simulink model "Rocket_Sim_1"  (R2021a)
settings: Solver=VariableStepAuto  StartTime=0.0  StopTime=550  MaxStep=0.001  RelTol=1e-3
values from neighbouring files (symbols this model uses):
  A = (pi*D^2)/4    (= 0.0490873852123)    [init_Rocket_Sim_1.m]    (also in old.m)
  A_drogue = (pi*D_drogue^2)/4    (= 0.125663706144)    [init_Rocket_Sim_1.m]    (also in old.m)
  A_e = pi*(De/2000)^2    (= 0.00196349540849)    [init_Rocket_Sim_1.m]
  A_para = (pi*D_para^2)/4    (= 1.13097335529)    [init_Rocket_Sim_1.m]    (also in old.m)
  Ae = pi*(De/2000)^2    (= 0.00196349540849)    [old.m]
  Cd = 0.5    [init_Rocket_Sim_1.m]    (also in old.m)
  Cd_para = 1.75    [init_Rocket_Sim_1.m]    (also in old.m)
  epsilon = 0.1    [init_Rocket_Sim_1.m]    (also in old.m)
  g = 9.81    [init_Rocket_Sim_1.m]    (also in old.m)
  m_dot = F/V_e    (= 1.78389398573)    [init_Rocket_Sim_1.m]    (also in old.m)
  m_dry = 50    [init_Rocket_Sim_1.m]    (also in old.m)
  m_Propellant = 118    [init_Rocket_Sim_1.m]    (also in old.m)
  p0 = 101325    [init_Rocket_Sim_1.m]    (also in old.m)
  R = 287    [init_Rocket_Sim_1.m]    (also in old.m)
  sigma = 5.6704e-8    (= 5.6704e-08)    [init_Rocket_Sim_1.m]    (also in old.m)
  V_e = g*Isp    (= 1962)    [init_Rocket_Sim_1.m]    (also in suvat_nonsense.m)
  Ve = g*Isp    (= 1962)    [old.m]
undefined symbols (not defined in the file or in its folder): ambient_temp, buck_cout, buck_cout_ESR, Buck_Ilim, buck_ind, buck_ind_ESR, DiscIntNeverNeededParam, Friction, ia, ib, Ion, J, Lithium, Lls, m, m0_fuel, m0_ox, m_f_dot, m_ox_dot, p, Rlim, Rs, supercap_max_voltage, supercap_val, thetam, Ts, Vref, wm
libraries: powerlib x18, electricdrivelib x3, pid_lib x2, powerlib_meascontrol x2, rllib x1
settings Model: SimulationMode=rapid-accelerator  Creator=marti  LastModifiedBy=Raihaan
settings SolverCC: MaxConsecutiveMinStep=5  AlgebraicLoopSolver=TrustRegion
settings DebuggingCC: SFMachineParentedDataDiag=warning

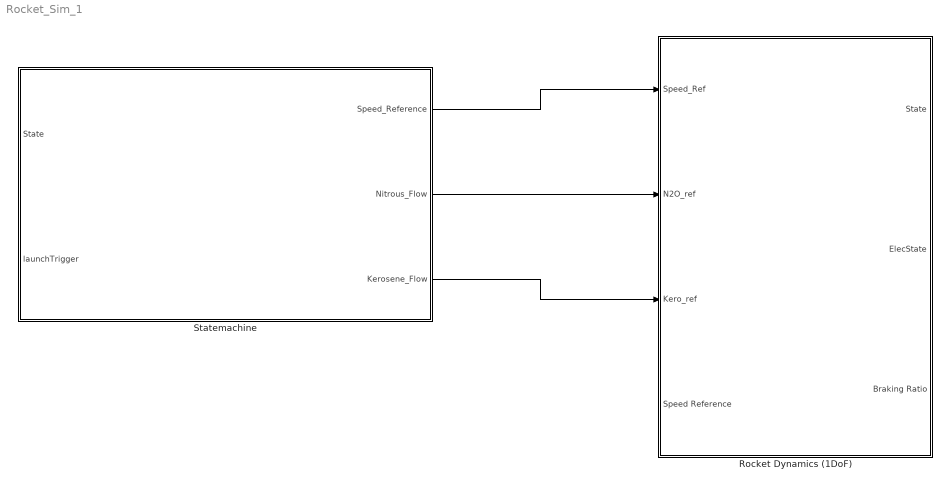
== system Rocket_Sim_1 ==
  Rocket Dynamics (1DoF) : Subsystem
      mask Display: image('$imagefile'); % Use "Edit Image" on toolstrip to change.
  Statemachine : Stateflow chart  TreatAsAtomicUnit=on
  wires:
  Statemachine/1(Speed_Reference) -> Rocket Dynamics (1DoF)/1(Speed_Ref)
  Statemachine/2(Nitrous_Flow) -> Rocket Dynamics (1DoF)/2(N2O_ref)
  Statemachine/3(Kerosene_Flow) -> Rocket Dynamics (1DoF)/3(Kero_ref)

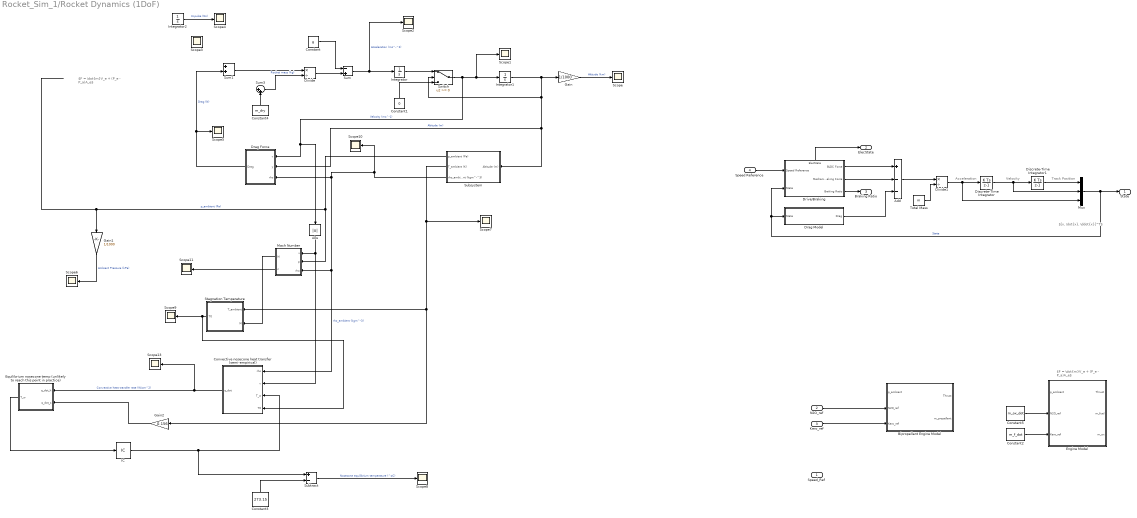
== system Rocket_Sim_1/Rocket Dynamics (1DoF) ==
  note: $F = \dot{m}V_e + (P_e - P_a)A_e$
  note: $[x, \dot{x}, \ddot{x}]^T$
  note: Acceleration
  note: Track Position
  note: Velocity
  note: $F = \dot{m}V_e + (P_e - P_a)A_e$
  Speed_Ref : Inport
  N2O_ref : Inport  Port=2
  Kero_ref : Inport  Port=3
  Speed Reference : Inport  Port=4
  Abs : Abs
  Add : Sum  Inputs=+--
  Bipropellant Engine Model : Subsystem
  Constant : Constant  Value=g
  Constant1 : Constant  Value=0
  Constant2 : Constant  Value=m_f_dot
  Constant3 : Constant  Value=273.15
  Constant4 : Constant  Value=m_dry
  Constant5 : Constant  Value=m_ox_dot
  Convective nosecone heat transfer (semi-empirical) : MATLAB Function  TreatAsAtomicUnit=on
  Discrete-Time Integrator : DiscreteIntegrator  SampleTime=-1  ICPrevOutput=DiscIntNeverNeededParam  ICPrevScaledInput=DiscIntNeverNeededParam
  Discrete-Time Integrator1 : DiscreteIntegrator  SampleTime=-1  LimitOutput=on  UpperSaturationLimit=500  LowerSaturationLimit=0  ICPrevOutput=DiscIntNeverNeededParam  ICPrevScaledInput=DiscIntNeverNeededParam
  Divide : Product  Inputs=*/
  Divide1 : Product  Inputs=*/
  Drag Force : Subsystem
  Drag Model : Subsystem
  Drive/Braking : Subsystem
      settings: PortSchema="{\"entries\":[{\"content\":{\"sides\":[{\"content\":{\"connectorIds\":[\"In1\",\"In2\"]},\"type\":\"ConnectorPlacement.EquallySpacedRectSide\",\"uuid\":\"aa5e316a-c8d3-4f13-ba46-5c76cbb2586c\"},{\"content\":{\"connectorIds\":[\"Out1\",\"Out2\",\"Out3\"],\"side\":\"RIGHT\"},\"type\":\"ConnectorPlacement.EquallySpacedRectSide\",\"uuid\":\"e4d6c32a-fd39-4302-8ddf-f7a48563407f\"},{\"content\":{\"connectorIds\":[\"Out4\"],\"side\":\"TOP\"},\"type\":\"ConnectorPlacement.EquallySpacedRectSide\",\"uuid\":\"af8256cd-30c6-4d91-a38a-bb87ecde33bd\"}]},\"type\":\"ConnectorPlacement.EquallySpacedConnector\",\"uuid\":\"2dd03fee-d1e4-4173-9dcd-593c38e6bfdd\"}],\"packageUris\":[\"http://schema.mathworks.com/mf0/Connector/R2020b\"],\"version\":\"1.0\"}"
  Engine Model : Subsystem
  Equilibrium nosecone temp (unlikely to reach this point in practice) : MATLAB Function  TreatAsAtomicUnit=on
  Gain : Gain  Gain=1/1000
  Gain1 : Gain  Gain=1/1000
  Gain2 : Gain  Gain=0.156
  IC : InitialCondition  Value=300
  Integrator : Integrator
  Integrator1 : Integrator
  Integrator2 : Integrator
  Mach Number : MATLAB Function  TreatAsAtomicUnit=on
  Mux : Mux  Inputs=3
  Scope{,1..11,13} (13 alike) : Scope
  Stagnation Temperature : MATLAB Function  TreatAsAtomicUnit=on
  Subsystem : Subsystem
  Subtract : Sum  Inputs=+-
  Sum : Sum  Inputs=-+
  Sum1 : Sum
  Sum3 : Sum  Inputs=|++
  Switch : Switch
  Total Mass : Constant  Value=m
  State : Outport
  ElecState : Outport  Port=2
  Braking Ratio : Outport  Port=3
  wires:
  Sum/1 -> Scope2/1, Integrator/1  "Acceleration (ms^-^2)"
  Subtract/1 -> Scope8/1  "Nosecone equilibrium temperature (^oC)"
  Constant4/1 -> Sum3/2
  Constant3/1 -> Subtract/2
  Integrator2/1 -> Scope4/1  "Impulse (Ns)"
  Gain1/1 -> Scope6/1  "Ambient Pressure (kPa)"
  Equilibrium nosecone temp (unlikely to reach this point in practice)/1(T_w) -> IC/1
  Integrator/1 -> Switch/1
  Gain2/1 -> Equilibrium nosecone temp (unlikely to reach this point in practice)/2(q_dot_s)
  Constant1/1 -> Switch/3
  Divide/1 -> Sum/2
  IC/1 -> Subtract/1, Convective nosecone heat transfer (semi-empirical)/3(T_w)
  ? -> Sum3/1  "Propellant mass (kg)"
  Abs/1 -> Convective nosecone heat transfer (semi-empirical)/2(v), Mach Number/1(v)
  Subsystem/1(p_ambient (Pa)) -> Mach Number/2(p), Gain1/1  "p_ambient (Pa)"
  Mach Number/1(M) -> Stagnation Temperature/2(M)
  Drag Force/1(Drag) -> Scope5/1, Sum1/2  "Drag (N)"
  Subsystem/3(rho_ambient (kgm^-^3)) -> Scope10/1, Convective nosecone heat transfer (semi-empirical)/1(rho), Mach Number/3(rho), Drag Force/3(rho)  "rho_ambient (kgm^-3)"
  Convective nosecone heat transfer (semi-empirical)/1(q_dot) -> Scope13/1, Equilibrium nosecone temp (unlikely to reach this point in practice)/1(q_dot_h)  "Convective heat transfer rate (W/cm^2)"
  ? -> Integrator2/1, Scope3/1, Sum1/1  "Thrust (N)"
  Switch/1 -> Drag Force/1(v), Abs/1, Scope1/1, Integrator1/1  "Velocity (ms^-1)"
  Sum1/1 -> Divide/1
  Integrator1/1 -> Switch/2, Drag Force/2(y), Subsystem/1(Altitude (m)), Gain/1  "Altitude (m)"
  Sum3/1 -> Divide/2  "Rocket mass (kg)"
  Mach Number/2(c) -> Scope11/1
  Subsystem/2(T_ambient (K)) -> Gain2/1, Stagnation Temperature/1(T_ambient), Scope7/1
  Gain/1 -> Scope/1  "Altitude (km)"
  Constant/1 -> Sum/1
  Stagnation Temperature/1(T0) -> Convective nosecone heat transfer (semi-empirical)/4(T0), Scope9/1
  Discrete-Time Integrator/1 -> Discrete-Time Integrator1/1, Mux/2
  Drag Model/1(Drag) -> Add/3
  Total Mass/1 -> Divide1/2
  Discrete-Time Integrator1/1 -> Mux/1
  Speed Reference/1 -> Drive/Braking/1(Speed Reference)
  Drive/Braking/4(ElecState) -> ElecState/1
  Drive/Braking/1(BLDC Force) -> Add/1
  Drive/Braking/3(Braking Ratio) -> Braking Ratio/1
  Mux/1 -> State/1, Drive/Braking/2(State), Drag Model/1(State)  "State"
  Drive/Braking/2(Mechanical Braking Force) -> Add/2
  Divide1/1 -> Discrete-Time Integrator/1, Mux/3
  Add/1 -> Divide1/1
  Kero_ref/1 -> Bipropellant Engine Model/3(Kero_ref)
  N2O_ref/1 -> Bipropellant Engine Model/2(N2O_ref)
  Constant5/1 -> Engine Model/2(N2O_ref)
  Constant2/1 -> Engine Model/3(Kero_ref)

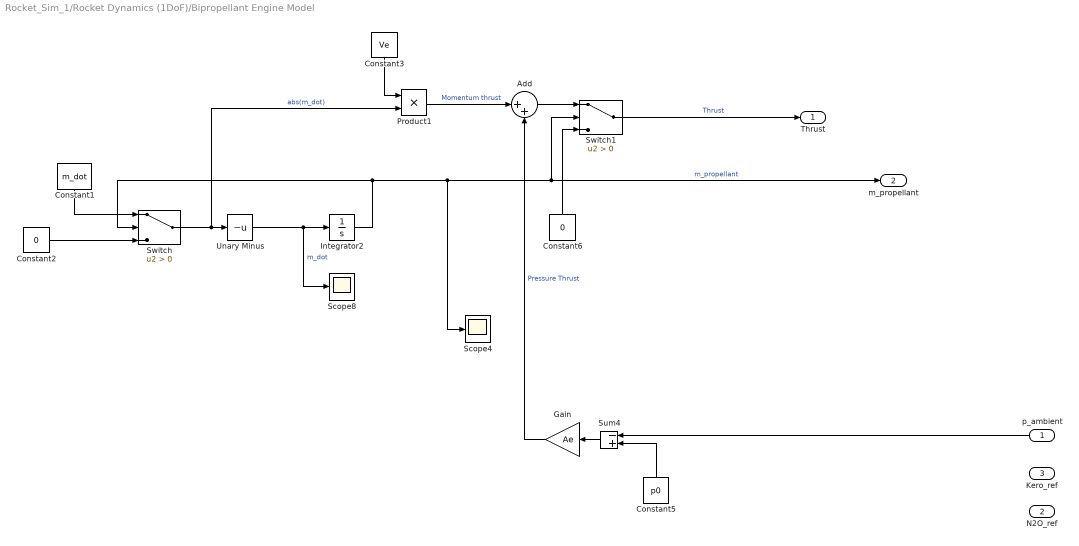
== system Rocket_Sim_1/Rocket Dynamics (1DoF)/Bipropellant Engine Model ==
  p_ambient : Inport
  N2O_ref : Inport  Port=2
  Kero_ref : Inport  Port=3
  Add : Sum  Inputs=|++
  Constant1 : Constant  Value=m_dot
  Constant2 : Constant  Value=0
  Constant3 : Constant  Value=Ve
  Constant5 : Constant  Value=p0
  Constant6 : Constant  Value=0
  Gain : Gain  Gain=Ae
  Integrator2 : Integrator  InitialCondition=m_Propellant
  Product1 : Product
  Scope4 : Scope
  Scope8 : Scope
  Sum4 : Sum  Inputs=-+
  Switch : Switch  Criteria=u2 > Threshold
  Switch1 : Switch  Criteria=u2 > Threshold
  Unary Minus : UnaryMinus
  Thrust : Outport
  m_propellant : Outport  Port=2
  wires:
  Unary Minus/1 -> Integrator2/1, Scope8/1  "m_dot"
  Constant6/1 -> Switch1/3
  Constant2/1 -> Switch/3
  Constant5/1 -> Sum4/2
  Add/1 -> Switch1/1
  Constant3/1 -> Product1/1
  Integrator2/1 -> m_propellant/1, Switch1/2, Scope4/1, Switch/2  "m_propellant"
  Switch/1 -> Product1/2, Unary Minus/1  "abs(m_dot)"
  Sum4/1 -> Gain/1
  Constant1/1 -> Switch/1
  Gain/1 -> Add/2  "Pressure Thrust"
  Switch1/1 -> Thrust/1  "Thrust"
  Product1/1 -> Add/1  "Momentum thrust"
  p_ambient/1 -> Sum4/1

== system Rocket_Sim_1/Rocket Dynamics (1DoF)/Drag Force ==
  v : Inport
  y : Inport  Port=2
  rho : Inport  Port=3
  Drag Force : MATLAB Function  TreatAsAtomicUnit=on
  Switch : Switch
  Unary Minus : UnaryMinus
  Drag : Outport
  wires:
  Drag Force/1(F_d) -> Switch/3, Unary Minus/1  "abs(F_d)"
  Switch/1 -> Drag/1  "F_d"
  v/1 -> Drag Force/1(v), Switch/2
  rho/1 -> Drag Force/3(rho)
  Unary Minus/1 -> Switch/1
  y/1 -> Drag Force/2(y)

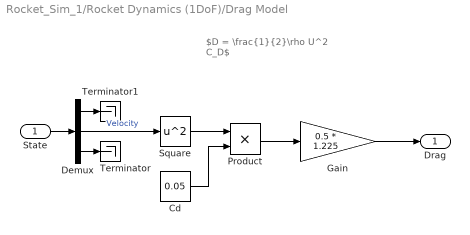
== system Rocket_Sim_1/Rocket Dynamics (1DoF)/Drag Model ==
  note: $D = \frac{1}{2}\rho U^2 C_D$
  State : Inport
  Cd : Constant  Value=0.05
  Demux : Demux  Outputs=3
  Gain : Gain  Gain=0.5 * 1.225
  Product : Product
  Square : Math  Operator=square  SaturateOnIntegerOverflow=on
  Terminator : Terminator
  Terminator1 : Terminator
  Drag : Outport
  wires:
  State/1 -> Demux/1
  Demux/3 -> Terminator/1
  Demux/1 -> Terminator1/1
  Demux/2 -> Square/1  "Velocity"
  Square/1 -> Product/1
  Cd/1 -> Product/2
  Product/1 -> Gain/1
  Gain/1 -> Drag/1

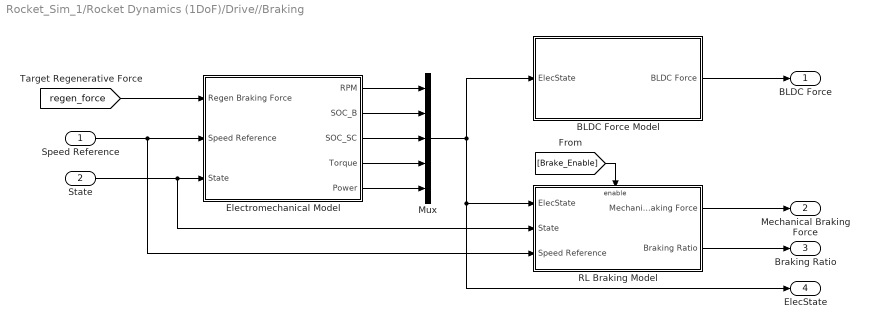
== system Rocket_Sim_1/Rocket Dynamics (1DoF)/Drive//Braking ==
  Speed Reference : Inport
  State : Inport  Port=2
  BLDC Force Model : Subsystem
  Electromechanical Model : Subsystem
  Mux : Mux  Inputs=5
  RL Braking Model : Subsystem
  BLDC Force : Outport
  Mechanical Braking Force : Outport  Port=2
  Braking Ratio : Outport  Port=3
  ElecState : Outport  Port=4
  wires:
  BLDC Force Model/1(BLDC Force) -> BLDC Force/1
  Speed Reference/1 -> Electromechanical Model/2(Speed Reference), RL Braking Model/3(Speed Reference)
  State/1 -> Electromechanical Model/3(State), RL Braking Model/2(State)
  [Brake_Enable] -> RL Braking Model/Enable
  RL Braking Model/2(Braking Ratio) -> Braking Ratio/1
  Electromechanical Model/1(RPM) -> Mux/1
  Electromechanical Model/2(SOC_B) -> Mux/2
  Electromechanical Model/3(SOC_SC) -> Mux/3
  Electromechanical Model/4(Torque) -> Mux/4
  Mux/1 -> ElecState/1, RL Braking Model/1(ElecState), BLDC Force Model/1(ElecState)
  [regen_force] -> Electromechanical Model/1(Regen Braking Force)
  RL Braking Model/1(Mechanical Braking Force) -> Mechanical Braking Force/1
  Electromechanical Model/5(Power) -> Mux/5

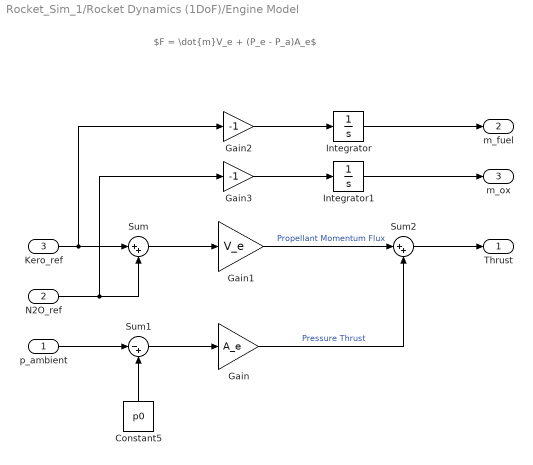
== system Rocket_Sim_1/Rocket Dynamics (1DoF)/Engine Model ==
  note: $F = \dot{m}V_e + (P_e - P_a)A_e$
  p_ambient : Inport
  N2O_ref : Inport  Port=2
  Kero_ref : Inport  Port=3
  Constant5 : Constant  Value=p0
  Gain : Gain  Gain=A_e
  Gain1 : Gain  Gain=V_e
  Gain2 : Gain  Gain=-1
  Gain3 : Gain  Gain=-1
  Integrator : Integrator  InitialCondition=m0_fuel
  Integrator1 : Integrator  InitialCondition=m0_ox
  Sum : Sum  Inputs=|++
  Sum1 : Sum  Inputs=|-+
  Sum2 : Sum  Inputs=|++
  Thrust : Outport
  m_fuel : Outport  Port=2
  m_ox : Outport  Port=3
  wires:
  Kero_ref/1 -> Gain2/1, Sum/1
  N2O_ref/1 -> Sum/2, Gain3/1
  Sum1/1 -> Gain/1
  Sum/1 -> Gain1/1
  Constant5/1 -> Sum1/2
  p_ambient/1 -> Sum1/1
  Gain1/1 -> Sum2/1  "Propellant Momentum Flux"
  Gain/1 -> Sum2/2  "Pressure Thrust"
  Sum2/1 -> Thrust/1
  Integrator/1 -> m_fuel/1
  Gain2/1 -> Integrator/1
  Integrator1/1 -> m_ox/1
  Gain3/1 -> Integrator1/1

== system Rocket_Sim_1/Rocket Dynamics (1DoF)/Subsystem ==
  Altitude (m) : Inport
  Earth Atmosphere Model : MATLAB Function  TreatAsAtomicUnit=on
  p_ambient (Pa) : Outport
  T_ambient (K) : Outport  Port=2
  rho_ambient (kgm^-^3) : Outport  Port=3
  wires:
  Earth Atmosphere Model/1(T) -> T_ambient (K)/1  "T_ambient (K)"
  Altitude (m)/1 -> Earth Atmosphere Model/1(y)
  Earth Atmosphere Model/2(p) -> p_ambient (Pa)/1
  Earth Atmosphere Model/3(rho) -> rho_ambient (kgm^-^3)/1

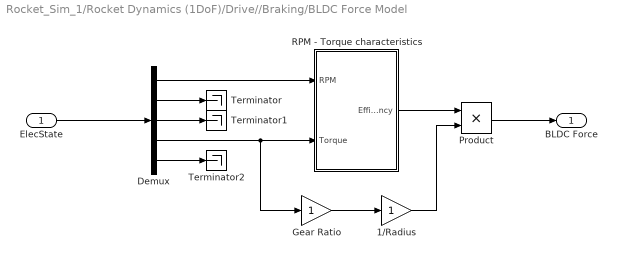
== system Rocket_Sim_1/Rocket Dynamics (1DoF)/Drive//Braking/BLDC Force Model ==
  ElecState : Inport
  1/Radius : Gain
  Demux : Demux  Outputs=5
  Gear Ratio : Gain
  Product : Product
  RPM - Torque characteristics : Subsystem
  Terminator : Terminator
  Terminator1 : Terminator
  Terminator2 : Terminator
  BLDC Force : Outport
  wires:
  Demux/1 -> RPM - Torque characteristics/1(RPM)
  Demux/3 -> Terminator1/1
  Gear Ratio/1 -> 1/Radius/1
  Demux/4 -> RPM - Torque characteristics/2(Torque), Gear Ratio/1
  Product/1 -> BLDC Force/1
  1/Radius/1 -> Product/2
  Demux/2 -> Terminator/1
  ElecState/1 -> Demux/1
  RPM - Torque characteristics/1(Efficiency) -> Product/1
  Demux/5 -> Terminator2/1

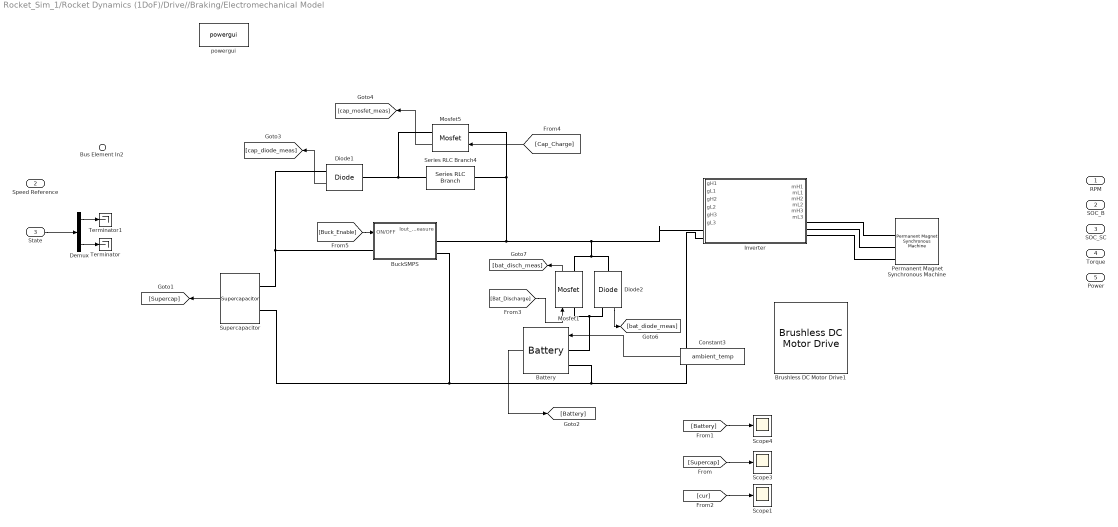
== system Rocket_Sim_1/Rocket Dynamics (1DoF)/Drive//Braking/Electromechanical Model ==
  Bus Element In2 : Inport  PortName=Regen Braking Force  Element=signal1
  Speed Reference : Inport  Port=2
  State : Inport  Port=3
  Battery : electricdrivelib/Extra Sources/Battery  BatType=Lithium-Ion  ShowTempParam=on  ThermalPreset="3.3V  2.3Ah  (LiFePO4)"  ShowAgeParam=off  NomV=3.3  NomQ=2.3  SOC=bat_initial_soc  Batt_Tr=30  PresetModel=off  MaxQ=2.3  MinV=2.475  FullV=3.748  Dis_rate=2.3  R=0.014  Normal_OP=2.25  expZone="[3.4788       0.113]"  current=[6.5 13 32.5]  Units=Time  Tci=20  NomT=25  T2=0  MaxQ2=2.208  FullV2=3.45  Normal_OP2=2.85  expZone2="[3.22       0.015]"  Rca=0.6  ti=1000  Dp=0  Neq0=0  Tsim=1e6  Ta1=25  Qeol=5.4*0.9  Reol=0.013333*1.2  Char_age=[2.3478, 3]  Dis_age=[2.3478, 10]  N1=1500  N2=10500  N3=1000  N4=1400  Ta2=45  N5=950
  Brushless DC Motor Drive1 : electricdrivelib/AC drives/Brushless DC Motor Drive  Rs=0.2  Lls=8.5e-3  Flat=120  MachineConstant=Flux linkage established by magnets (V.s)  FluxCst=0.175  VoltageCst=146.6077  TorqueCst=1.4  ia=0  ib=0  J=0.089  Friction=0.005  p=4  wm=0  thetam=0  Rsnb_rec=10e3  Csnb_rec=20e-9  Ron_rec=1e-3  Vf_rec=1.3  cap_bus=2000e-6  Rbrake=8  fbrake=4000  activationVoltage=320  shutdownVoltage=310  deviceType=IGBT / Diodes  Ron_inv=1e-3  Vf_inv=0.8  Vfd_inv=0.8  Tf=1e-6  Tt=2e-6  Tf_GTO=10e-6  Tt_GTO=20e-6  Rsnb_inv=5000  Csnb_inv=inf  regulationType=Speed regulation  Acc=1000  Dec=-1000  kp_sc=3.3  ki_sc=300  fc_sc=285  Tsc=140e-6  Tmin=-17.8  Tmax=17.8  h=0.01  freq_max=20e3  Tvect=20e-6  zeta=0.99  Trd=0.13/5  K1=3000  K2=-49500  baseSampleTime=2e-06  outputBusMode=Multiple output buses  busLabels=off  sensorless=off  MechanicalLoad=Torque Tm  modelDetailLevel=Detailed  driveType=AC7  AverageValue=off
      settings: SourceProductBaseCode=PS
  BuckSMPS : Subsystem
  Constant3 : Constant  Value=ambient_temp
  Demux : Demux  Outputs=3
  Diode1 : powerlib/Power Electronics/Diode  Ron=0.001  Lon=0  Vf=Vf_Diode  IC=0  UseSnubber=0  Rs=500  Cs=250e-9  Measurements=on
  Diode2 : powerlib/Power Electronics/Diode  Ron=0.001  Lon=0  Vf=Vf_Diode  IC=0  UseSnubber=0  Rs=500  Cs=250e-9  Measurements=on
  Inverter : Subsystem
  Mosfet1 : powerlib/Power Electronics/Mosfet  Ron=Pch_Ron  Lon=0  Rd=0.01  Vfd=Pch_Vd  IC=0  Rs=1e9  Cs=inf  Measurements=on
  Mosfet5 : powerlib/Power Electronics/Mosfet  Ron=Pch_Ron  Lon=0  Rd=0.01  Vfd=Pch_Vd  IC=0  Rs=1e9  Cs=inf  Measurements=on
  Permanent Magnet Synchronous Machine : powerlib/Machines/Permanent Magnet Synchronous Machine  NbPhases=3  FluxDistribution=Trapezoidal  RotorType=Round  MechanicalLoad=Torque Tm  PresetModel=No  ShowDetailedParameters=on  MeasurementBus=off  Resistance=Rs  Inductance=Lls  dqInductances=[8.5e-3,8.5e-3]  La=0.000835  MachineConstant=Flux linkage established by magnets (V.s)  Flux=0.175  VoltageCst=146.6077  TorqueCst=1.4  Flat=Flat  Mechanical=[J,Friction,p]  PolePairs=4  InitialConditions=[wm,thetam,ia,ib]  InitialConditions5ph=[0 0 0 0 0 0]  RefAngle=90 degrees behind phase A axis (modified Park)  IterativeDiscreteModel=Trapezoidal non iterative  TsBlock=-1  TsPowergui=0
  Scope1 : Scope
  Scope3 : Scope
  Scope4 : Scope
  Series RLC Branch4 : powerlib/Elements/Series RLC Branch  LConnTagsString=__new0  RConnTagsString=__new0  BranchType=R  Resistance=Rlim  Inductance=1e-3  SetiL0=off  InitialCurrent=0  Capacitance=1e-6  Setx0=off  InitialVoltage=0  Measurements=Branch voltage and current
  Supercapacitor : electricdrivelib/Extra Sources/Supercapacitor  C=supercap_val  Rdc=supercap_ESR  Voltage=supercap_max_voltage  Ns=18  Np=1  Vinit=supercap_initial_voltage  Temp=ambient_temp  PresetModel=off  EstParam=off  Nc=1  r=1e-9  epsilon=6.0208e-10  Ich=10  Vstern="[0.161  2.7  7.8]"  Self_dis=on  Ioc=10  Vself="[48  47.8  47.06  44.65]"  demandeplot=off  I="[10  20 100  500]"  Units=sec  Vmax=0  If=0  deltaV=0  alpha=0  sec=0
      settings: SourceProductBaseCode=PS
  Terminator : Terminator
  Terminator1 : Terminator
  powergui : powerlib/powergui  Priority=1  SimulationMode=Discrete  SampleTime=Ts  frequency=60  Iterations=50  frequencyindice=0  Pbase=100e6  ErrMax=1e-4  UnitsV=kV  UnitsW=MW  buscounter=0  FunctionMessages=off  echomessages=off  EnableUseOfTLC=off  CurrentSourceSwitches=off  DisableSnubberDevices=off  DisableRonSwitches=off  DisableVfSwitches=off  DisplayEquations=off  AutomaticDiscreteSolvers=off  SolverType=Tustin/Backward Euler (TBE)  Interpol=off  ExternalGateDelay=off  methode=off  Ts=100  x0status=blocks  SPID=on  SwTol=0  HookPort=off  NonlinearTolerance=1e-4  nMaxIteration=100  ContinueOnMaxIteration=off  RestoreLinks=warning  ResistiveCurrentMeasurement=off  Frange=[0:2:500]  Ylog=off  Xlog=on  ShowGrid=off  save=off  variable=ZData  structure=0  ZoomFFT=off  StartTime=0.0  cycles=1  DisplayStyle=1  fundamental=60  FreqAxis=off  MaxFrequency=1000  frequencyindicesteady=1  RmsSteady=1  display=off
  RPM : Outport
  SOC_B : Outport  Port=2
  SOC_SC : Outport  Port=3
  Torque : Outport  Port=4
  Power : Outport  Port=5
  wires:
  [Battery] -> Scope4/1
  [cur] -> Scope1/1
  Diode2/1 -> [bat_diode_meas]
  [Cap_Charge] -> Mosfet5/1
  Mosfet5/1 -> [cap_mosfet_meas]
  Mosfet1/1 -> [bat_disch_meas]
  Battery/1 -> [Battery]
  Diode1/1 -> [cap_diode_meas]
  Constant3/1 -> Battery/1
  Supercapacitor/1 -> [Supercap]
  [Supercap] -> Scope3/1
  Demux/1 -> Terminator1/1
  Demux/3 -> Terminator/1
  State/1 -> Demux/1
  [Bat_Discharge] -> Mosfet1/1
  [Buck_Enable] -> BuckSMPS/1(ON/OFF)
  connections:
  Series RLC Branch4/LConn1 -- Mosfet1/RConn1 -- Diode2/LConn1 -- Inverter/LConn1 -- BuckSMPS/RConn1 -- Mosfet5/LConn1
  Diode1/RConn1 -- BuckSMPS/LConn1 -- Supercapacitor/LConn1
  Inverter/LConn2 -- BuckSMPS/RConn2 -- Supercapacitor/LConn2 -- Battery/LConn2
  Mosfet1/LConn1 -- Diode2/RConn1 -- Battery/LConn1
  Diode1/LConn1 -- Series RLC Branch4/RConn1 -- Mosfet5/RConn1
  Inverter/RConn3 -- Permanent Magnet Synchronous Machine/LConn3
  Permanent Magnet Synchronous Machine/LConn1 -- Inverter/RConn1
  Inverter/RConn2 -- Permanent Magnet Synchronous Machine/LConn2

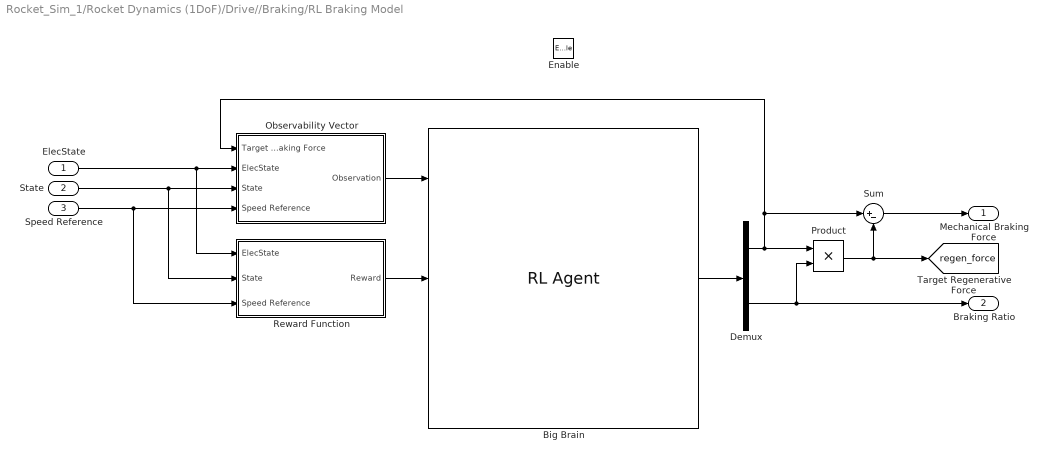
== system Rocket_Sim_1/Rocket Dynamics (1DoF)/Drive//Braking/RL Braking Model ==
  ElecState : Inport
  State : Inport  Port=2
  Speed Reference : Inport  Port=3
  Enable : EnablePort
  Big Brain : rllib/RL Agent  Agent=agentObj  ExternalActionAsInput=off  ProvideCumRwd=off  TreatAsDirectFeedthrough=on  mask(RL Agent){}
      mask Display: image('$imagefile'); % Use "Edit Image" on toolstrip to change.
  Demux : Demux  Outputs=2
  Observability Vector : Subsystem
      mask Display: image('$imagefile'); % Use "Edit Image" on toolstrip to change.
  Product : Product
  Reward Function : Subsystem
      mask Display: image('$imagefile'); % Use "Edit Image" on toolstrip to change.
  Sum : Sum  Inputs=|+-
  Mechanical Braking Force : Outport
  Braking Ratio : Outport  Port=2
  tag scope: regen_force=global
  wires:
  State/1 -> Reward Function/2(State), Observability Vector/3(State)
  Reward Function/1(Reward) -> Big Brain/2
  Observability Vector/1(Observation) -> Big Brain/1
  ElecState/1 -> Reward Function/1(ElecState), Observability Vector/2(ElecState)
  Product/1 -> Sum/2, [regen_force]
  Big Brain/1 -> Demux/1
  Demux/1 -> Product/1, Observability Vector/1(Target Braking Force), Sum/1
  Demux/2 -> Product/2, Braking Ratio/1
  Speed Reference/1 -> Reward Function/3("Speed Reference "), Observability Vector/4(Speed Reference)
  Sum/1 -> Mechanical Braking Force/1

== system Rocket_Sim_1/Rocket Dynamics (1DoF)/Drive//Braking/BLDC Force Model/RPM - Torque characteristics ==
  RPM : Inport
  Torque : Inport  Port=2
  Gain : Gain
  Efficiency : Outport
  wires:
  RPM/1 -> Gain/1
  Gain/1 -> Efficiency/1

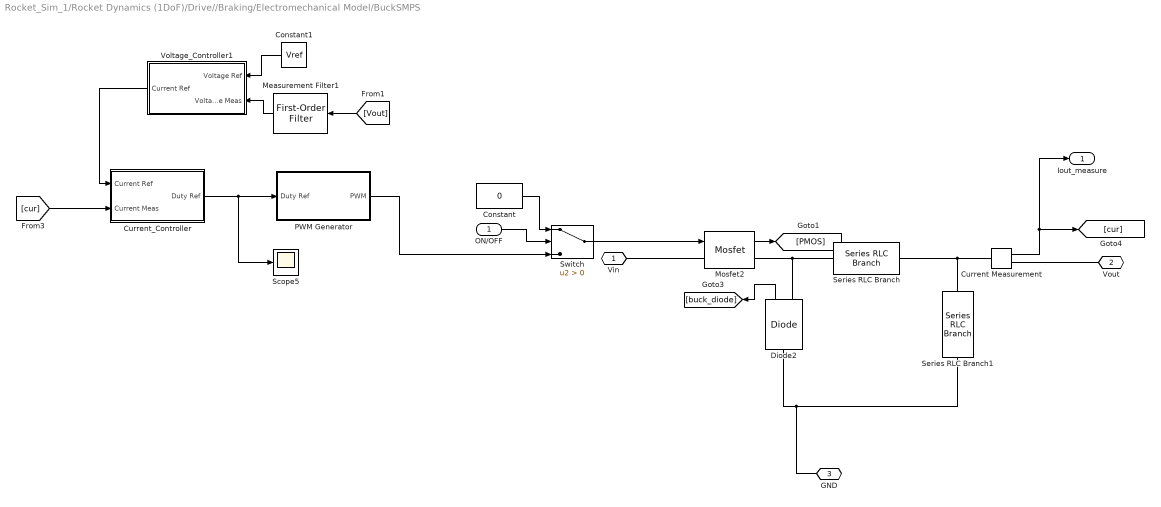
== system Rocket_Sim_1/Rocket Dynamics (1DoF)/Drive//Braking/Electromechanical Model/BuckSMPS ==
  ON/OFF : Inport
  Constant : Constant  Value=0
  Constant1 : Constant  Value=Vref
  Current Measurement : powerlib/Measurements/Current Measurement  PhasorSimulation=off  OutputType=Complex  PSBequivalent=0
  Current_Controller : Subsystem
  Diode2 : powerlib/Power Electronics/Diode  Ron=0.001  Lon=0  Vf=Vf_Diode  IC=0  UseSnubber=0  Rs=500  Cs=250e-9  Measurements=on
  Measurement Filter1 : powerlib_meascontrol/Filters/First-Order Filter  FilterType=Lowpass  Tc=10000*2.2e-9  Ts=0  Initialize=on  Vac_Init=[0, 0, 0]  Vdc_Init=0  PlotResponse=off  FreqRange="[0,  100e3,  100]"
  Mosfet2 : powerlib/Power Electronics/Mosfet  Ron=Pch_Ron  Lon=0  Rd=0.01  Vfd=Pch_Vd  IC=0  Rs=1e9  Cs=inf  Measurements=on
  PWM Generator : Subsystem
  Scope5 : Scope
  Series RLC Branch : powerlib/Elements/Series RLC Branch  LConnTagsString=__new0  RConnTagsString=__new0  BranchType=RL  Resistance=buck_ind_ESR  Inductance=buck_ind  SetiL0=off  InitialCurrent=0  Capacitance=1e-6  Setx0=off  InitialVoltage=0  Measurements=None
  Series RLC Branch1 : powerlib/Elements/Series RLC Branch  LConnTagsString=__new0  RConnTagsString=__new0  BranchType=RC  Resistance=buck_cout_ESR  Inductance=1e-3  SetiL0=off  InitialCurrent=0  Capacitance=buck_cout  Setx0=off  InitialVoltage=0  Measurements=Branch voltage and current
  Switch : Switch  Criteria=u2 > Threshold
  Voltage_Controller1 : Subsystem
  Vin : PMIOPort  Side=Left
  Vout : PMIOPort  Port=2  Side=Right
  GND : PMIOPort  Port=3  Side=Right
  Iout_measure : Outport
  wires:
  [cur] -> Current_Controller/2(Current Meas)
  PWM Generator/1(PWM) -> Switch/3
  Current Measurement/1 -> Iout_measure/1, [cur]
  Current_Controller/1(Duty Ref) -> Scope5/1, PWM Generator/1(Duty Ref)
  Mosfet2/1 -> [PMOS]
  Diode2/1 -> [buck_diode]
  [Vout] -> Measurement Filter1/1
  Measurement Filter1/1 -> Voltage_Controller1/2(Voltage Meas)
  Constant1/1 -> Voltage_Controller1/1(Voltage Ref)
  Voltage_Controller1/1(Current Ref) -> Current_Controller/1(Current Ref)
  ON/OFF/1 -> Switch/2
  Switch/1 -> Mosfet2/1
  Constant/1 -> Switch/1
  connections:
  Mosfet2/RConn1 -- Diode2/RConn1 -- Series RLC Branch/LConn1
  Series RLC Branch/RConn1 -- Current Measurement/LConn1 -- Series RLC Branch1/LConn1
  Current Measurement/RConn1 -- Vout/RConn1
  Mosfet2/LConn1 -- Vin/RConn1
  Series RLC Branch1/RConn1 -- Diode2/LConn1 -- GND/RConn1

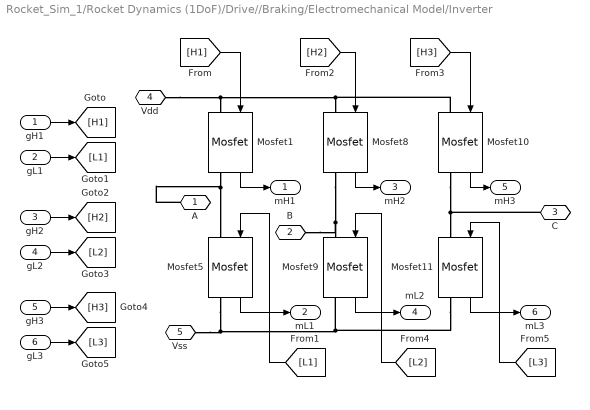
== system Rocket_Sim_1/Rocket Dynamics (1DoF)/Drive//Braking/Electromechanical Model/Inverter ==
  gH1 : Inport
  gL1 : Inport  Port=2
  gH2 : Inport  Port=3
  gL2 : Inport  Port=4
  gH3 : Inport  Port=5
  gL3 : Inport  Port=6
  Mosfet{1,5,8..11} (6 alike) : powerlib/Power Electronics/Mosfet  Ron=0.1  Lon=0  Rd=0.01  Vfd=0  IC=0  Rs=1e5  Cs=inf  Measurements=on
  A : PMIOPort  Side=Right
  B : PMIOPort  Port=2  Side=Right
  C : PMIOPort  Port=3  Side=Right
  Vdd : PMIOPort  Port=4  Side=Left
  Vss : PMIOPort  Port=5  Side=Left
  mH1 : Outport
  mL1 : Outport  Port=2
  mH2 : Outport  Port=3
  mL2 : Outport  Port=4
  mH3 : Outport  Port=5
  mL3 : Outport  Port=6
  wires:
  Mosfet11/1 -> mL3/1
  [L2] -> Mosfet9/1
  Mosfet5/1 -> mL1/1
  [H3] -> Mosfet10/1
  gL2/1 -> [L2]
  [H2] -> Mosfet8/1
  Mosfet9/1 -> mL2/1
  Mosfet10/1 -> mH3/1
  Mosfet1/1 -> mH1/1
  Mosfet8/1 -> mH2/1
  [L1] -> Mosfet5/1
  gL3/1 -> [L3]
  gH3/1 -> [H3]
  gL1/1 -> [L1]
  gH2/1 -> [H2]
  gH1/1 -> [H1]
  [H1] -> Mosfet1/1
  [L3] -> Mosfet11/1
  connections:
  Mosfet5/RConn1 -- Vss/RConn1 -- Mosfet11/RConn1 -- Mosfet9/RConn1
  Vdd/RConn1 -- Mosfet8/LConn1 -- Mosfet10/LConn1 -- Mosfet1/LConn1
  Mosfet1/RConn1 -- Mosfet5/LConn1 -- A/RConn1
  Mosfet10/RConn1 -- Mosfet11/LConn1 -- C/RConn1
  Mosfet8/RConn1 -- B/RConn1 -- Mosfet9/LConn1

== system Rocket_Sim_1/Rocket Dynamics (1DoF)/Drive//Braking/RL Braking Model/Observability Vector ==
  Target Braking Force : Inport
  ElecState : Inport  Port=2
  State : Inport  Port=3
  Speed Reference : Inport  Port=4
  Mux : Mux
  Observation : Outport
  wires:
  Mux/1 -> Observation/1
  Target Braking Force/1 -> Mux/1
  ElecState/1 -> Mux/2
  State/1 -> Mux/3
  Speed Reference/1 -> Mux/4

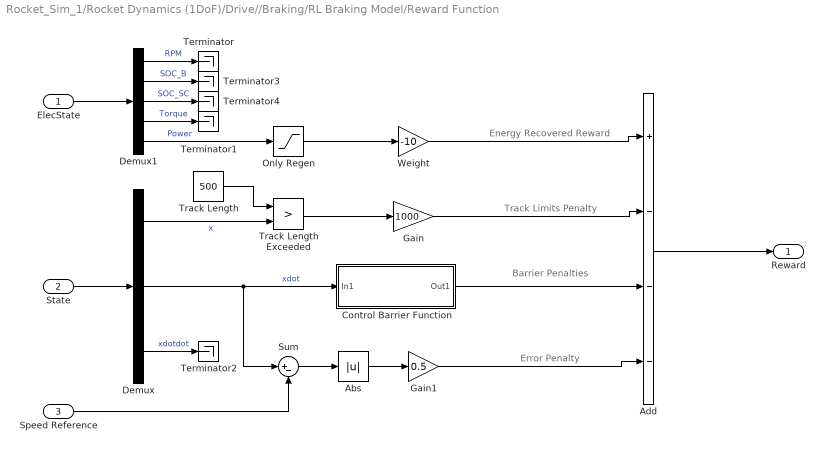
== system Rocket_Sim_1/Rocket Dynamics (1DoF)/Drive//Braking/RL Braking Model/Reward Function ==
  note: Barrier Penalties
  note: Track Limits Penalty
  note: Error Penalty
  note: Energy Recovered Reward
  ElecState : Inport
  State : Inport  Port=2
  "Speed Reference " : Inport  Port=3
  Abs : Abs
  Add : Sum  Inputs=+---
  Control Barrier Function : Subsystem
  Demux : Demux  Outputs=3
  Demux1 : Demux  Outputs=5
  Gain : Gain  Gain=1000
  Gain1 : Gain  Gain=0.5
  Only Regen : Saturate  UpperLimit=0  LowerLimit=-inf
  Sum : Sum  Inputs=|+-
  Terminator{,1..4} (5 alike) : Terminator
  Track Length : Constant  Value=500
  Track Length Exceeded : RelationalOperator  Operator=>  OutDataTypeStr=boolean  RndMeth=Simplest
  Weight : Gain  Gain=-10
  Reward : Outport
  wires:
  Demux1/3 -> Terminator4/1  "SOC_SC"
  Demux/1 -> Track Length Exceeded/2  "x"
  Abs/1 -> Gain1/1
  Sum/1 -> Abs/1
  Track Length Exceeded/1 -> Gain/1
  Gain1/1 -> Add/4
  Gain/1 -> Add/2
  "Speed Reference "/1 -> Sum/2
  Weight/1 -> Add/1
  Track Length/1 -> Track Length Exceeded/1
  Demux/2 -> Sum/1, Control Barrier Function/1(In1)  "xdot"
  Control Barrier Function/1(Out1) -> Add/3
  Only Regen/1 -> Weight/1
  State/1 -> Demux/1
  Demux/3 -> Terminator2/1  "xdotdot"
  Demux1/1 -> Terminator/1  "RPM"
  ElecState/1 -> Demux1/1
  Demux1/4 -> Terminator1/1  "Torque"
  Demux1/5 -> Only Regen/1  "Power"
  Add/1 -> Reward/1
  Demux1/2 -> Terminator3/1  "SOC_B"

== system Rocket_Sim_1/Rocket Dynamics (1DoF)/Drive//Braking/Electromechanical Model/BuckSMPS/Current_Controller ==
  Current Ref : Inport
  Current Meas : Inport  Port=2
  Discrete PID Controller : pid_lib/PID Controller  Controller=PID  Form=Parallel  TimeDomain=Discrete-time  UseExternalTs=off  SampleTime=1/1000  IntegratorMethod=Forward Euler  FilterMethod=Forward Euler  ControllerParametersSource=internal  P=0.02512  I=39.4  D=0  UseFilter=off  N=100  TunerSelectOption=Transfer Function Based (PID Tuner App)  InitialConditionSource=internal  InitialConditionForIntegrator=0  InitialConditionForFilter=0  DifferentiatorICPrevScaledInput=0  ExternalReset=none  TrackingMode=off  Kt=1  LimitOutput=off  SatLimitsSource=internal  UpperSaturationLimit=inf  LowerSaturationLimit=-inf  LinearizeAsGain=off  AntiWindupMode=none  Kb=1  POutMin=[]  POutMax=[]  IOutMin=[]  IOutMax=[]  DOutMin=[]  DOutMax=[]  NOutMin=[]  NOutMax=[]  SumOutMin=[]  SumOutMax=[]  SaturationOutMin=[]  SaturationOutMax=[]  PParamMin=[]  PParamMax=[]  IParamMin=[]  IParamMax=[]  DParamMin=[]  DParamMax=[]  NParamMin=[]  NParamMax=[]  KbParamMin=[]  KbParamMax=[]  KtParamMin=[]  KtParamMax=[]  KbOutMin=[]  KbOutMax=[]  KtOutMin=[]  KtOutMax=[]  IntegratorOutMin=[]  IntegratorOutMax=[]  FilterOutMin=[]  FilterOutMax=[]  SumI1OutMin=[]  SumI1OutMax=[]  SumI2OutMin=[]  SumI2OutMax=[]  SumI3OutMin=[]  SumI3OutMax=[]  SumI4OutMin=[]  SumI4OutMax=[]  SumDOutMin=[]  SumDOutMax=[]  DifferentiatorOutMin=[]  DifferentiatorOutMax=[]  FilterDiffOutCoefMin=[]  FilterDiffOutCoefMax=[]  ReciprocalOutMin=[]  ReciprocalOutMax=[]  SumDenOutMin=[]  SumDenOutMax=[]  SumNumOutMin=[]  SumNumOutMax=[]  DivideOutMin=[]  DivideOutMax=[]  UdiffTsProdOutMin=[]  UdiffTsProdOutMax=[]  NTsProdOutMin=[]  NTsProdOutMax=[]  UintegralTsProdOutMin=[]  UintegralTsProdOutMax=[]  UngainTsProdOutMin=[]  UngainTsProdOutMax=[]  IntegratorContinuousStateAttributes=''  IntegratorStateMustResolveToSignalObject=off  IntegratorRTWStateStorageClass=Auto  FilterContinuousStateAttributes=''  FilterStateMustResolveToSignalObject=off  FilterRTWStateStorageClass=Auto  ParallelPVariant=InternalParameters  IdealPVariant=Disabled  IVariant=InternalParameters  DVariant=InternalParameters  IntegratorVariant=Discrete  SatVariant=Disabled  AWVariant=Passthrough  PCopyVariant=Disabled  TRVariant=Disabled  FdbkBlocksVariant=Forward  IdealPFdbkVariant=Disabled  SatFdbkVariant=Disabled  DerivativeFilterVariant=Differentiator  NVariant=Passthrough  NCopyVariant=Disabled_SignalSpec  FilterICVariant=InternalICsDifferentiator  IntegratorICVariant=InternalICs  ExternalResetVariant=Disabled  TRSumVariant=Passthrough  SumFdbkVariant=Disabled  SumVariant=Sum_PID  TsampFilterVariant=InternalTs  TsampNgainVariant=Passthrough  TsampIntegralVariant=Passthrough  ExternalSaturationOutDataTypeStr=Inherit: Same as second input
  Saturation : Saturate  UpperLimit=0.98  LowerLimit=0.02
  Subtract : Sum  Inputs=+-
  Duty Ref : Outport
  wires:
  Subtract/1 -> Discrete PID Controller/1
  Saturation/1 -> Duty Ref/1
  Current Meas/1 -> Subtract/2
  Discrete PID Controller/1 -> Saturation/1
  Current Ref/1 -> Subtract/1

== system Rocket_Sim_1/Rocket Dynamics (1DoF)/Drive//Braking/Electromechanical Model/BuckSMPS/PWM Generator ==
  note: This is a PWM generator using a sawtooth waveform and comparator.
      |
      | The sawtooth function gives an output +/-1 and we need to be in the range 0-1 and therefore needs offsetting.
  Duty Ref : Inport
  Add : Sum
  Constant : Constant
  Gain : Gain  Gain=0.5
  Relational Operator : RelationalOperator  Operator=>  OutDataTypeStr=boolean  RndMeth=Simplest
  Sawtooth Generator : powerlib_meascontrol/Pulse & Signal Generators/Sawtooth Generator  Freq=62500  Phase=180  Ts=Ts
  PWM : Outport
  wires:
  Duty Ref/1 -> Relational Operator/1
  Relational Operator/1 -> PWM/1
  Constant/1 -> Add/2
  Add/1 -> Gain/1
  Sawtooth Generator/1 -> Add/1
  Gain/1 -> Relational Operator/2

== system Rocket_Sim_1/Rocket Dynamics (1DoF)/Drive//Braking/Electromechanical Model/BuckSMPS/Voltage_Controller1 ==
  Voltage Ref : Inport
  Voltage Meas : Inport  Port=2
  Discrete PID Controller1 : pid_lib/PID Controller  Controller=PID  Form=Parallel  TimeDomain=Discrete-time  UseExternalTs=off  SampleTime=1/1000  IntegratorMethod=Forward Euler  FilterMethod=Forward Euler  ControllerParametersSource=internal  P=0.05024  I=15.78  D=0  UseFilter=off  N=100  TunerSelectOption=Transfer Function Based (PID Tuner App)  InitialConditionSource=internal  InitialConditionForIntegrator=0  InitialConditionForFilter=0  DifferentiatorICPrevScaledInput=0  ExternalReset=none  TrackingMode=off  Kt=1  LimitOutput=off  SatLimitsSource=internal  UpperSaturationLimit=inf  LowerSaturationLimit=-inf  LinearizeAsGain=off  AntiWindupMode=none  Kb=1  POutMin=[]  POutMax=[]  IOutMin=[]  IOutMax=[]  DOutMin=[]  DOutMax=[]  NOutMin=[]  NOutMax=[]  SumOutMin=[]  SumOutMax=[]  SaturationOutMin=[]  SaturationOutMax=[]  PParamMin=[]  PParamMax=[]  IParamMin=[]  IParamMax=[]  DParamMin=[]  DParamMax=[]  NParamMin=[]  NParamMax=[]  KbParamMin=[]  KbParamMax=[]  KtParamMin=[]  KtParamMax=[]  KbOutMin=[]  KbOutMax=[]  KtOutMin=[]  KtOutMax=[]  IntegratorOutMin=[]  IntegratorOutMax=[]  FilterOutMin=[]  FilterOutMax=[]  SumI1OutMin=[]  SumI1OutMax=[]  SumI2OutMin=[]  SumI2OutMax=[]  SumI3OutMin=[]  SumI3OutMax=[]  SumI4OutMin=[]  SumI4OutMax=[]  SumDOutMin=[]  SumDOutMax=[]  DifferentiatorOutMin=[]  DifferentiatorOutMax=[]  FilterDiffOutCoefMin=[]  FilterDiffOutCoefMax=[]  ReciprocalOutMin=[]  ReciprocalOutMax=[]  SumDenOutMin=[]  SumDenOutMax=[]  SumNumOutMin=[]  SumNumOutMax=[]  DivideOutMin=[]  DivideOutMax=[]  UdiffTsProdOutMin=[]  UdiffTsProdOutMax=[]  NTsProdOutMin=[]  NTsProdOutMax=[]  UintegralTsProdOutMin=[]  UintegralTsProdOutMax=[]  UngainTsProdOutMin=[]  UngainTsProdOutMax=[]  IntegratorContinuousStateAttributes=''  IntegratorStateMustResolveToSignalObject=off  IntegratorRTWStateStorageClass=Auto  FilterContinuousStateAttributes=''  FilterStateMustResolveToSignalObject=off  FilterRTWStateStorageClass=Auto  ParallelPVariant=InternalParameters  IdealPVariant=Disabled  IVariant=InternalParameters  DVariant=InternalParameters  IntegratorVariant=Discrete  SatVariant=Disabled  AWVariant=Passthrough  PCopyVariant=Disabled  TRVariant=Disabled  FdbkBlocksVariant=Forward  IdealPFdbkVariant=Disabled  SatFdbkVariant=Disabled  DerivativeFilterVariant=Differentiator  NVariant=Passthrough  NCopyVariant=Disabled_SignalSpec  FilterICVariant=InternalICsDifferentiator  IntegratorICVariant=InternalICs  ExternalResetVariant=Disabled  TRSumVariant=Passthrough  SumFdbkVariant=Disabled  SumVariant=Sum_PID  TsampFilterVariant=InternalTs  TsampNgainVariant=Passthrough  TsampIntegralVariant=Passthrough  ExternalSaturationOutDataTypeStr=Inherit: Same as second input
  Saturation1 : Saturate  UpperLimit=Buck_Ilim  LowerLimit=0
  Subtract1 : Sum  Inputs=+-
  Current Ref : Outport
  wires:
  Saturation1/1 -> Current Ref/1
  Subtract1/1 -> Discrete PID Controller1/1
  Voltage Ref/1 -> Subtract1/1
  Discrete PID Controller1/1 -> Saturation1/1
  Voltage Meas/1 -> Subtract1/2

== system Rocket_Sim_1/Rocket Dynamics (1DoF)/Drive//Braking/RL Braking Model/Reward Function/Control Barrier Function ==
  In1 : Inport
  Out1 : Outport
  wires:
  In1/1 -> Out1/1

== matlab function Rocket_Sim_1/Rocket Dynamics (1DoF)/Drag Force/Drag Force ==
  data: v input; y input; F_d output; rho input; Cd parameter; A parameter; Cd_para parameter; A_para parameter; A_drogue parameter
function F_d = fcn(v, y, rho, Cd, A, Cd_para, A_para, A_drogue)
if v > -20
    F_d = 0.5*A*rho*Cd*v^2; %Calculate drag force for rocket on ascent
else
    if y > 1000
        F_d = 0.5*A*rho*Cd*v^2 + 0.5*A_drogue*rho*Cd_para*v^2; %Calculate drag force for rocket + drogue parachute on descent
    elseif y >800
        F_d = 0.5*A*rho*Cd*v^2 + 0.5*(A_para/2)*rho*Cd_para*v^2; %Calculate drag force for rocket + reefed parachute on descent
    else
        F_d = 0.5*A*rho*Cd*v^2 + 0.5*A_para*rho*Cd_para*v^2; %Calculate drag force for rocket + parachute on descent
    end
end

== matlab function Rocket_Sim_1/Rocket Dynamics (1DoF)/Subsystem/Earth Atmosphere Model ==
  data: y input; T output; p output; rho output; p0 parameter; R parameter; g parameter
function [T, p, rho] = fcn(y, p0, R, g)
%Using NASA atmosphere model for pressure: https://www.grc.nasa.gov/www/k-12/airplane/atmosmet.html
%And "definition of standard temperatures at different altitudes" for temperature: http://www.ambrsoft.com/CalcPhysics/Altitude/altitude.htm

T0 = 288.15; %Temperature at y = 0
L0 = -0.0065; %Rate of change of temperature with height (in K/m)

T1 = 216.65;
p1 = p0*(T1/T0)^(-g/(R*L0));

T2 = T1;
L2 = 0.001;
p2 = p1*exp(g*(11000 - 20000)/(R*T2));

T3 = 228.65;
L3 = 0.0028;
p3 = p2*(T3/T2)^(-g/(R*L2));

T4 = 270.65;
p4 = p3*(T4/T3)^(-g/(R*L3));

T5 = T4;
L5 = -0.0028;
p5 = p4*exp(g*(47000 - 51000)/(R*T4));

T6 = 214.65;
L6 = -0.002;
p6 = p5*(T6/T5)^(-g/(R*L5));

T7 = 186.95;
p7 = p6*(T7/T6)^(-g/(R*L6));

T8 = T7;
L8 = 0.004;
p8 = p7*exp(g*(84852 - 90000)/(R*T7));

%Work out atmospheric temperature in K
if y < 11000 %Troposphere (0 to 1)
    T = T0 + L0*y;
    p = p0*(T/T0)^(-g/(R*L0));
elseif y >= 11000 && y < 20000 %Tropopause (1 to 2)
    T = T1;
    p = p1*exp(g*(11000 - y)/(R*T1));
elseif y >= 20000 && y < 32000 %Lower stratosphere (2 to 3)
    T = T2 + L2*(y - 20000);
    p = p2*(T/T2)^(-g/(R*L2));
elseif y >= 32000 && y < 47000 %Upper stratosphere (3 to 4)
    T = T3 + L3*(y - 32000);
    p = p3*(T/T3)^(-g/(R*L3));
elseif y >= 47000 && y < 51000 %Stratopause (4 to 5)
    T = T4;
    p = p4*exp(g*(47000 - y)/(R*T4));
elseif y >= 51000 && y < 71000 %Lower mesosphere (5 to 6)
    T = T5 + L5*(y - 51000);
    p = p5*(T/T5)^(-g/(R*L5));
elseif y >= 71000 && y < 84852 %Upper mesosphere (6 to 7)
    T = T6 + L6*(y - 71000);
    p = p6*(T/T6)^(-g/(R*L6));
elseif y >= 84852 && y < 90000 %Mesopause (7 to 8)
    T = T7;
    p = p7*exp(g*(84852 - y)/(R*T7));
else %Thermosphere
    T = T8 + L8*(y - 90000);
    p = p8*(T/T8)^(-g/(R*L8));
end


%NASA atmosphere model for pressure
%if y < 11000 %Troposphere
 %   p = 101290 * (T/288.08)^5.256; %Calculate air pressure in Pa
%elseif y >= 11000 && y < 25000 %Lower Stratosphere
 %   p = 22650 * exp(1.73 - 0.000157*y); %Calculate air pressure in Pa
%else %Upper Stratosphere
 %   p = 2488*((T/216.6)^(-11.388)); %Calculate air pressure in Pa
%end
rho = p/(0.2869*T*1000);

== matlab function Rocket_Sim_1/Rocket Dynamics (1DoF)/Mach Number ==
  data: v input; M output; p input; rho input; c output; gamma parameter
function [M, c] = fcn(v, p, rho, gamma)
c = sqrt(gamma*p/rho); %calculate local speed of sound using equation for an ideal gas
M = v/c; %Calculate mach number from local speed of sound and velocity

== matlab function Rocket_Sim_1/Rocket Dynamics (1DoF)/Stagnation Temperature ==
  data: T_ambient input; T0 output; M input; gamma parameter
function T0 = fcn(T_ambient, M, gamma)
%See ICLR wiki article for details: https://wiki.imperial.ac.uk/display/IRW/Estimating+Thermal+Loads+on+Rockets
T0 = T_ambient*(1+((gamma-1)/2)*M^2); %Calculate stagnation temperature in K

== matlab function Rocket_Sim_1/Rocket Dynamics (1DoF)/Convective nosecone heat transfer (semi-empirical) ==
  data: q_dot output; rho input; v input; T_w input; T0 input; r_n parameter
function q_dot = fcn(rho, v, T_w, T0, r_n)
N = 0.5;
M = 3;
g_w = T_w/T0;
C = 1.83e-8 * (1/sqrt(r_n))*(1 - g_w);
q_dot = C*(rho^N)*(v^M);

== matlab function Rocket_Sim_1/Rocket Dynamics (1DoF)/Equilibrium nosecone temp (unlikely to reach this point in practice) ==
  data: q_dot_h input; q_dot_s input; T_w output; epsilon parameter; sigma parameter
function T_w = fcn(q_dot_h, q_dot_s, epsilon, sigma)
%epsilon is the surface emissivity of the nosecone, sigma is the
%Stefan-Boltzmann constant
T_w = ((q_dot_h + q_dot_s)/(epsilon*sigma))^0.25;

== stateflow chart Rocket_Sim_1/Statemachine ==
  state Flight [parallel]
    settings: executionOrder=1
    state Straight
      entry:
      send(Straight, Dynamics);
    state Bend
      entry:
      send(Bend, Dynamics);
    state Finish
      entry:
      send(Finish, Dynamics);
    (default) -> Straight
    Bend -> Straight : [State(1) > 300]
    Straight -> Bend [order 2] : [State(1) > 200]
    Straight -> Finish [order 1] : [State(1) >= 500]
  state Nitrous [parallel]
    settings: executionOrder=2
    state Idle
      entry:
      Buck_Enable = 0;
      Cap_Charge = 0;
    state Charging
      entry:
      Cap_Charge = 1;
    state Discharging
      entry:
      Cap_Charge = 0;
      Buck_Enable = 1;
    (default) -> Nitrous.Idle
    Nitrous.Discharging -> Nitrous.Idle [order 1] : IDLE
    Nitrous.Charging -> Nitrous.Idle [order 1] : IDLE
    Nitrous.Idle -> Nitrous.Charging [order 1] : CHARGE
    Nitrous.Idle -> Nitrous.Discharging [order 2] : DISCHARGE
    Nitrous.Charging -> Nitrous.Discharging [order 2] : DISCHARGE
    Nitrous.Discharging -> Nitrous.Charging [order 2] : CHARGE{Buck_Enable = 0;}
  state Kerosene [parallel]
    settings: executionOrder=3
    state Idle
      entry:
      Bat_Discharge = 0;
    state Charging
      entry:
      Bat_Discharge = 1;
    state Discharging
      entry:
      Bat_Discharge = 1;
    (default) -> Kerosene.Idle
    Kerosene.Charging -> Kerosene.Idle [order 1] : IDLE
    Kerosene.Discharging -> Kerosene.Idle [order 1] : IDLE
    Kerosene.Idle -> Kerosene.Charging [order 1] : CHARGE
    Kerosene.Idle -> Kerosene.Discharging [order 2] : DISCHARGE
    Kerosene.Charging -> Kerosene.Discharging [order 2] : DISCHARGE
    Kerosene.Discharging -> Kerosene.Charging [order 2] : CHARGE
  state Dynamics [parallel]
    settings: executionOrder=4
    state Idle
      entry:
      Preflight();
      Speed_Reference = 0;
      Brake_Enable = 0;
    state Shutdown
      entry:
      send(IDLE, SC);
      send(IDLE, Kerosene);
      PostFlight();
    state Braking
      state HardBraking
        entry:
        Speed_Reference = 0;
        send(CHARGE, SC)
      state SoftBraking
        entry:
        Speed_Reference = 100;
        send(CHARGE, SC)
      (default) -> (junction 28)
      (junction 28) -> HardBraking [order 2]
      (junction 28) -> (junction 53) [order 1] : Bend
      (junction 53) -> SoftBraking
    state Pushing
      state Boosted
        entry:
        send(DISCHARGE, SC);
        send(DISCHARGE, Kerosene);
      state Nominal
        entry:
        send(IDLE, SC);
      (default) -> Boosted
      Boosted -> Nominal : [ElecState(3) < 0.05]
      Nominal -> Boosted : [ElecState(3) > 0.5]
    (default) -> Dynamics.Idle
    Dynamics.Idle -> Pushing : [launchTrigger==1]{Speed_Reference = 120}
    Braking -> Shutdown [order 1] : Finish
    (junction 115) -> Braking
    Pushing -> Braking : [BrakePredictor(State)]{Brake_Enable = 1;
        | Buck_Enable = 0}
    (junction 114) -> (junction 115) [order 1] : [ElecState(2) > 0.95]
        | {send(IDLE, Kerosene);}
    (junction 114) -> Braking [order 2]
    Braking -> Pushing [order 2] : [BrakePredictor(State)]{Brake_Enable = 0}
    Braking -> (junction 114) [order 3] : [ElecState(3) > 0.95]
        | {send{IDLE, SC};
        |  send(CHARGE, Kerosene);}
  data: State function_input; State input; Speed_Reference output; Nitrous_Flow output; launchTrigger input; Kerosene_Flow output
  function Preflight:
    | function Preflight
    |  
    | an%% Simulation parameters
    | clear
    | 
    | Ts = 0.1;                          % Sample time for the model
    | Fsw = 62000;                        % Switching frequency of the PWM
    | Run_Time = 5;                      % Amount of time to simulate
    | Vref = 3.3;                         % Initialise.
    | Buck_Ilim = 3;                      % Current limit in the buck converter
    | 
    | %% Circuit parameters
    | % BUCK bits
    | buck_cout = 1000e-6;
    | buck_cout_ESR = 0.1114;
    | buck_ind = 100e-6;
    | buck_ind_ESR = 25e-3;
    | 
    | % MOSFETS and diodes
    | Pch_Ron = 0.136;                    %MOSFET On-state resistance
    | Pch_Vd = 1.1;                       %MOSFET parallel diode voltage
    | Vf_Diode = 0.7;                     %Diode Forward Voltage
    | 
    | % Three-phase source
    | source_rin = 0.8929;
    | source_ind = 16.58e-3;
    | source_Vline = 5;
    | 
    | % Supercap
    | supercap_val = 99.5;
    | supercap_ESR = 8.9e-3;
    | supercap_max_voltage = 48;
    |  
    | Rlim = 100e3;
    | 
    | 
    | supercap_initial_voltage = 40;
    | bat_initial_soc = 50; % percent
    | bat_initial_temp = 20; % degrees
    | ambient_temp = 22;
    | 
    | 
    | % %% S1: NORMAL MODE (battery supplies motor)
    | % cap_charging_mosfet = 0;
    | % bat_disch_mosfet = 1;
    | % buck_switch = 0;
    | % 
    | % supercap_initial_voltage = 40;
    | % bat_initial_soc = 50; % percent
    | % bat_initial_temp = 20; % degrees
    | % ambient_temp = 22;
    | % 
    | % sim("generator_model",Run_Time);
    | % %% S2: ACCELERATION MODE (supercapacitor assists battery)
    | % cap_charging_mosfet = 0;
    | % bat_disch_mosfet = 1;
    | % buck_switch = 1;
    | % 
    | % supercap_initial_voltage = 40;
    | % bat_initial_soc = 50; % percent
    | % bat_initial_temp = 20; % degrees
    | % Vref = 3.3; % reference voltage for the buck: same as battery voltage.
    | % ambient_temp = 22;
    | % 
    | % sim("motor_model",Run_Time);
    | % %% S3: REGEN BRAKING SUPERCAP FLOW (motor charges supercap)
    | % cap_charging_mosfet = 1;
    | % bat_disch_mosfet = 0;
    | % buck_switch = 0;
    | % 
    | % supercap_initial_voltage = 40;
    | % bat_initial_soc = 50; % percent
    | % bat_initial_temp = 20; % degrees
    | % ambient_temp = 22;
    | % 
    | % % sim("generator_model",Run_Time);
    | % %% S4: REGEN BRAKING BATTERY FLOW
    | % cap_charging_mosfet = 0;
    | % bat_disch_mosfet = 1;
    | % buck_switch = 0;
    | % 
    | % supercap_initial_voltage = 40;
    | % bat_initial_soc = 50; % percent
    | % bat_initial_temp = 20; % degrees
    | % ambient_temp = 22;
    | % 
    | % % sim("generator_model",Run_Time);
  function BrakePredictor(State):
    | function BrakePredictor(State)
  function PostFlight:
    | function PostFlight
